simulink model "NCO_32"  (R2023a)
settings: Solver=VariableStepAuto  StartTime=0.0  StopTime=100  RelTol=1e-3
values from neighbouring files (symbols this model uses):
  bhi = fir2(79,f,mi)    [fir2my.m]
libraries: dsphdlfiltering2 x1, dsphdlsigops2 x1
settings Model: Creator=31651  LastModifiedBy=31651
settings OptimizationCC: BlockReduction=off  ConditionallyExecuteInputs=off  DefaultParameterBehavior=Inlined
settings DebuggingCC: AlgebraicLoopMsg=error
settings HardwareCC: ProdBitPerPointer=32  ProdBitPerSizeT=32  ProdBitPerPtrDiffT=32  ProdLargestAtomicFloat=None  ProdIntDivRoundTo=Undefined  ProdEndianess=Unspecified  ProdWordSize=32  ProdHWDeviceType=ASIC/FPGA->ASIC/FPGA  TargetBitPerPointer=64  TargetBitPerSizeT=64  TargetBitPerPtrDiffT=64  TargetLongLongMode=on  TargetIntDivRoundTo=Zero  TargetEndianess=LittleEndian  TargetWordSize=64  TargetHWDeviceType=Custom Processor->MATLAB Host Computer  ProdEqTarget=off

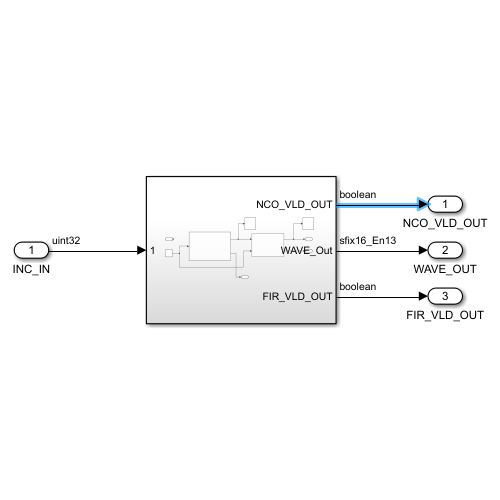
[thumbnail: Simulink's stored preview of the top-level diagram]
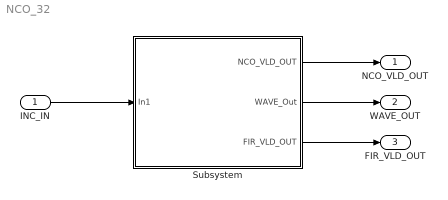
== system NCO_32 ==
  INC_IN : Inport  OutDataTypeStr=uint32
  Subsystem : Subsystem
  NCO_VLD_OUT : Outport  VectorParamsAs1DForOutWhenUnconnected=off
  WAVE_OUT : Outport  Port=2  VectorParamsAs1DForOutWhenUnconnected=off
  FIR_VLD_OUT : Outport  Port=3  VectorParamsAs1DForOutWhenUnconnected=off
  wires:
  INC_IN/1 -> Subsystem/1(In1)
  Subsystem/1(NCO_VLD_OUT) -> NCO_VLD_OUT/1
  Subsystem/2(WAVE_Out) -> WAVE_OUT/1
  Subsystem/3(FIR_VLD_OUT) -> FIR_VLD_OUT/1

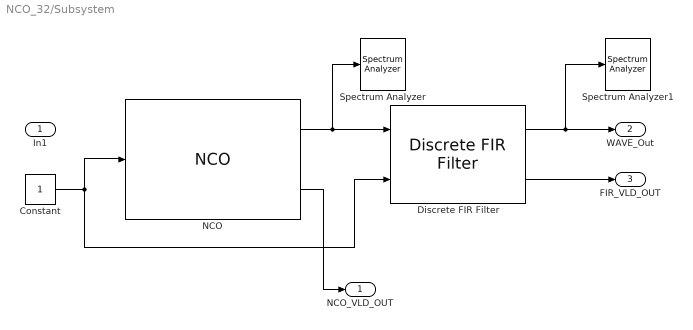
== system NCO_32/Subsystem ==
  In1 : Inport
  Constant : Constant  OutDataTypeStr=boolean  SampleTime=0.001
  Discrete FIR Filter : dsphdlfiltering2/Discrete FIR Filter  NumeratorSource=Property  Numerator=bhi  NumeratorPrototype=[]  FilterStructure=Direct form systolic  SerializationOption=Minimum number of cycles between valid input samples  NumCycles=2  NumberOfMultipliers=2  SimulateUsing=Code generation  roundingMode=Floor  overflowMode=off  CoefficientsDataTypeStr=Inherit: Same word length as input  OutputDataTypeStr=Inherit: Same word length as input  ResetInputPort=off  HDLGlobalReset=off
  NCO : dsphdlsigops2/NCO  PhaseIncrementSource=Property  PhaseIncrement=65535  PhaseOffsetSource=Property  PhaseOffset=0  DitherSource=Property  NumDitherBits=4  SamplesPerFrame=1  LUTCompress=off  ResetAction=off  Waveform=Sine  PhasePort=off  SimulateUsing=Code generation  AccumulatorWL=16  PhaseQuantization=on  NumQuantizerAccumulatorBits=12  OutputDataType=Binary point scaling  OutputWL=16  OutputFL=14
      settings: LibrarySourceBlock=dsphdlsrcs2/NCO
  Spectrum Analyzer : SpectrumAnalyzer  WindowPosition=[368.000000,182.000000,800.000000,500.000000,]  ScopeFrameLocation=window  SampleRateSource=Property  SampleRate=44.1e3  PlotAsTwoSidedSpectrum=off  FrequencyScale=Log  FrequencySpan=Start and stop frequencies  StartFrequency=20  StopFrequency=20e3  YLimits=[-85.99401411,40.26392201]  ColorLimits=[-20 80]  DefaultConfigurationName=spbscopes.SpectrumAnalyzerBlockCfg  IsFrequencyInputMode=0  FrequencyVectorPort=0  FrequencyVectorFromPort=0  FrequencyInputRBWPort=0  FrequencyInputRBWFromPort=0
  Spectrum Analyzer1 : SpectrumAnalyzer  WindowPosition=[368.000000,182.000000,800.000000,500.000000,]  Visible=on  ScopeFrameLocation=window  SampleRateSource=Property  SampleRate=44.1e3  PlotAsTwoSidedSpectrum=off  FrequencyScale=Log  FrequencySpan=Start and stop frequencies  StartFrequency=20  StopFrequency=20e3  YLimits=[-86.14603274,40.2176747]  ColorLimits=[-20 80]  DefaultConfigurationName=spbscopes.SpectrumAnalyzerBlockCfg  IsFrequencyInputMode=0  FrequencyVectorPort=0  FrequencyVectorFromPort=0  FrequencyInputRBWPort=0  FrequencyInputRBWFromPort=0
  NCO_VLD_OUT : Outport  VectorParamsAs1DForOutWhenUnconnected=off
  WAVE_Out : Outport  Port=2  VectorParamsAs1DForOutWhenUnconnected=off
  FIR_VLD_OUT : Outport  Port=3  VectorParamsAs1DForOutWhenUnconnected=off
  wires:
  Constant/1 -> NCO/1, Discrete FIR Filter/2
  NCO/2 -> NCO_VLD_OUT/1
  NCO/1 -> Spectrum Analyzer/1, Discrete FIR Filter/1
  Discrete FIR Filter/1 -> Spectrum Analyzer1/1, WAVE_Out/1
  Discrete FIR Filter/2 -> FIR_VLD_OUT/1
